simulink model "Fig117"  (R2014a)
settings: Solver=FixedStepDiscrete  StartTime=0.0  StopTime=.05  FixedStep=1e-3  RelTol=1e-3
libraries: commutil2 x2, commrandsrc2 x1
settings Model: Creator=Silage  LastModifiedBy=Silage

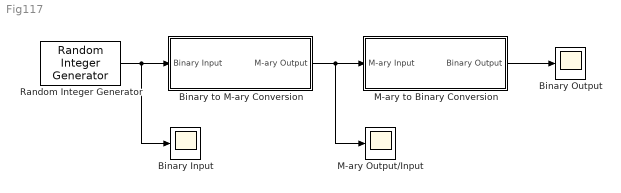
== system Fig117 ==
  Binary Input : Scope
      settings: YMin=-1  YMax=2
  Binary Output : Scope
      settings: YMin=-1  YMax=2  SaveName=ScopeData2
  Binary to M-ary Conversion : Subsystem
  M-ary Output/Input : Scope
      settings: YMin=-1  YMax=8
  M-ary to Binary Conversion : Subsystem
  Random Integer Generator : commrandsrc2/Random Integer Generator  mul=2  seed=37  Ts=1e-3  frameBased=off  sampPerFrame=1  orient=off  outDataType=double
  wires:
  Random Integer Generator/1 -> Binary Input/1, Binary to M-ary Conversion/1(Binary Input)
  Binary to M-ary Conversion/1("M-ary Output ") -> M-ary to Binary Conversion/1(M-ary Input), M-ary Output/Input/1
  M-ary to Binary Conversion/1(Binary Output) -> Binary Output/1

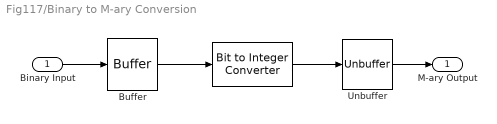
== system Fig117/Binary to M-ary Conversion ==
  Binary Input : Inport
  " " : commutil2/Bit to Integer Converter  nbits=3  bitOrder=MSB first  signedOutputValues=Unsigned  outDtype=Inherit via internal rule  outDtypeSigned=Inherit via internal rule
  Buffer : Buffer  N=3  TreatMby1Signals=One channel
  Unbuffer : Unbuffer  SampleBasedProcessing=Same as frame based
  "M-ary Output " : Outport
  wires:
  Binary Input/1 -> Buffer/1
  Buffer/1 -> " "/1
  " "/1 -> Unbuffer/1
  Unbuffer/1 -> "M-ary Output "/1

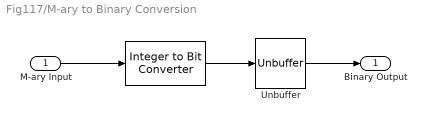
== system Fig117/M-ary to Binary Conversion ==
  M-ary Input : Inport
  " " : commutil2/Integer to Bit Converter  nbits=3  signedInputValues=Unsigned  bitOrder=MSB first  outDtype=Inherit via internal rule
  Unbuffer : Unbuffer  SampleBasedProcessing=Same as frame based
  Binary Output : Outport
  wires:
  " "/1 -> Unbuffer/1
  M-ary Input/1 -> " "/1
  Unbuffer/1 -> Binary Output/1
